simulink model "evse_power"  (R2023b)
settings: Solver=VariableStepAuto  StartTime=0.0  StopTime=10.0  RelTol=1e-3
libraries: fl_lib x6, nesl_utility x4
settings Model: Creator=dawid  LastModifiedBy=dawid
settings OptimizationCC: BooleanDataType=off

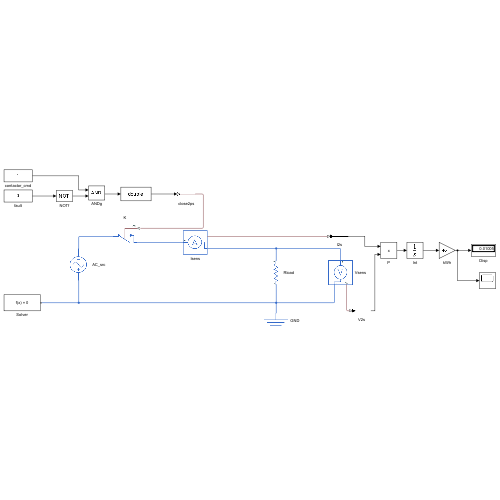
[thumbnail: Simulink's stored preview of the top-level diagram]
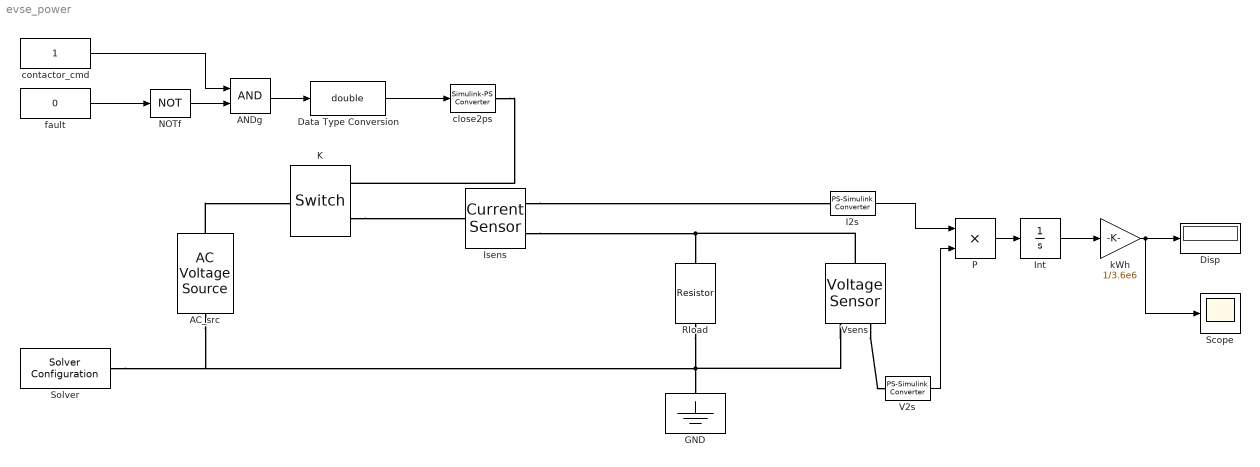
== system evse_power ==
  AC_src : fl_lib/Electrical/Electrical Sources/AC Voltage Source  amp=325 V  shift=0 deg  frequency=50 Hz  omega=0 rad/s
  ANDg : Logic  AllPortsSameDT=off  OutDataTypeStr=boolean
  Data Type Conversion : DataTypeConversion  OutDataTypeStr=double  SaturateOnIntegerOverflow=off  RndMeth=Floor
  Disp : Display
  GND : fl_lib/Electrical/Electrical Elements/Electrical Reference
  I2s : nesl_utility/PS-Simulink Converter  PhysicalDomain=network_engine_domain  SubClassName=ps_output  LeftPortType=input  RightPortType=output  PseudoPeriodic=off  Frequencies=[]  VectorFormat=inherit  Unit=inherit  AffineConversion=off
  Int : Integrator
  Isens : fl_lib/Electrical/Electrical Sensors/Current Sensor
  K : fl_lib/Electrical/Electrical Elements/Switch  R_closed=0.01 Ohm  G_open=1e-8 1/Ohm  Threshold=0.5  i_specify=off  i_priority=None  i=0 A  i_nominal_specify=off  i_nominal_unit=A  i_nominal_value=1  v_specify=off  v_priority=None  v=0 V  v_nominal_specify=off  v_nominal_unit=V  v_nominal_value=1
  NOTf : Logic  Operator=NOT  AllPortsSameDT=off  OutDataTypeStr=boolean
  P : Product
  Rload : fl_lib/Electrical/Electrical Elements/Resistor  R=14.4 Ohm  i_specify=off  i_priority=None  i=0 A  i_nominal_specify=off  i_nominal_unit=A  i_nominal_value=1  v_specify=off  v_priority=None  v=0 V  v_nominal_specify=off  v_nominal_unit=V  v_nominal_value=1
  Scope : Scope
  Solver : nesl_utility/Solver Configuration  PhysicalDomain=network_engine_domain  SubClassName=solver  LeftPortType=input  RightPortType=generic  Tones=[]  Harmonics=[]  SimulateNoise=off  Profile=off  UseLocalSampling=off  EnableSwitchedLinearOptims=on  FrequencyDomain=off  UseCCode=off  RelTol=0.001  AbsTol=0.001  MinStep=1e-09  ToWorkspace=off  RevertToSquareIcSolve=off  NumHomotopyIterations=100  PhasorMode=off  PhasorModeNumHarmonics=1  ConsistencySolver=NEWTON_XTOL_AFTER_FTOL  IndexReductionMethod=DerivativeReplacement  DoDC=off  ResidualTolerance=1e-09  ConsistencyTolSource=GLOBAL  ConsistencyAbsTol=0.001  ConsistencyRelTol=0.001  ConsistencyTolFactor=0.001  UseLocalSolver=off  LocalSolverChoice=NE_BACKWARD_EULER_ADVANCER  ResolveIndetEquations=on  FunctionEvalNumThread=1  LocalSolverSampleTime=0.001  DoFixedCost=off  MaxNonlinIter=3  MaxModeIter=2  ComputeImpulses=off  ImpulseIterations=2  LinearAlgebra=auto  LinearAlgebraNumThread=0  EquationFormulation=NE_TIME_EF  DelaysMemoryBudget=1024  AutomaticFiltering=on  FilteringTimeConstant=0.001  PartitionStorageMethod=AS_NEEDED  PartitionMemoryBudget=1024  PartitionMethod=ROBUST  MultibodyUseLocalSolver=off  MultibodyLocalSolverChoice=ODE1  MultibodyLocalSolverSampleTime=0.001
  V2s : nesl_utility/PS-Simulink Converter  PhysicalDomain=network_engine_domain  SubClassName=ps_output  LeftPortType=input  RightPortType=output  PseudoPeriodic=off  Frequencies=[]  VectorFormat=inherit  Unit=inherit  AffineConversion=off
  Vsens : fl_lib/Electrical/Electrical Sensors/Voltage Sensor
  close2ps : nesl_utility/Simulink-PS Converter  PhysicalDomain=network_engine_domain  SubClassName=ps_input  LeftPortType=input  RightPortType=output  PseudoPeriodic=off  Frequencies=[]  NoiseDistribution=none  NoiseParameters=[]  Unit=1  AffineConversion=off  FilteringAndDerivatives=provide  SimscapeFilterOrder=1  InputFilterTimeConstant=0.001  UdotUserProvided=0
  contactor_cmd : Constant
  fault : Constant  Value=0
  kWh : Gain  Gain=1/3.6e6
  wires:
  contactor_cmd/1 -> ANDg/1
  fault/1 -> NOTf/1
  NOTf/1 -> ANDg/2
  I2s/1 -> P/1
  V2s/1 -> P/2
  P/1 -> Int/1
  Int/1 -> kWh/1
  kWh/1 -> Disp/1, Scope/1
  ANDg/1 -> Data Type Conversion/1
  Data Type Conversion/1 -> close2ps/1
  connections:
  AC_src/RConn1 -- K/LConn1
  Rload/RConn1 -- AC_src/LConn1 -- Solver/RConn1 -- GND/LConn1 -- Vsens/RConn2
  Vsens/LConn1 -- Isens/RConn2 -- Rload/LConn1
  close2ps/RConn1 -- K/RConn1
  Isens/RConn1 -- I2s/LConn1
  Vsens/RConn1 -- V2s/LConn1
  K/RConn2 -- Isens/LConn1
